simulink model "vf_controlled_3_phase_squirrel_cage"  (R2024a)
settings: Solver=VariableStepAuto  StartTime=0.0  StopTime=5  RelTol=1e-3
libraries: spsControlledVoltageSourceLib x3, simulink x2, spsAsynchronousMachineSIUnitsLib x1, spsGroundLib x1, sps_lib x1
settings Model: Creator=baileyraven  LastModifiedBy=baileyraven
settings SolverCC: ZeroCrossAlgorithm=Adaptive
settings OptimizationCC: ReuseModelBlockBuffer=off
settings DebuggingCC: IgnoredZcDiagnostic=none
settings RTWCC: GPUComputeCapability=3.5

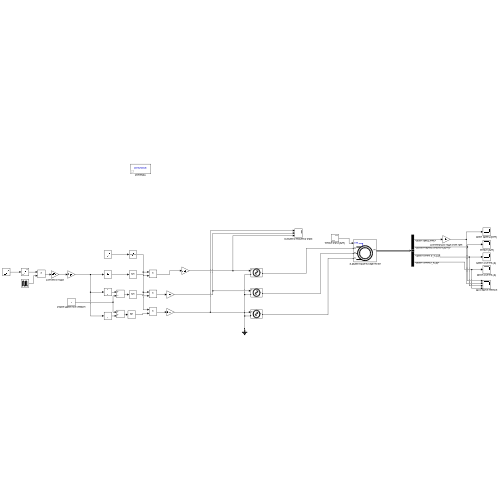
[thumbnail: Simulink's stored preview of the top-level diagram]
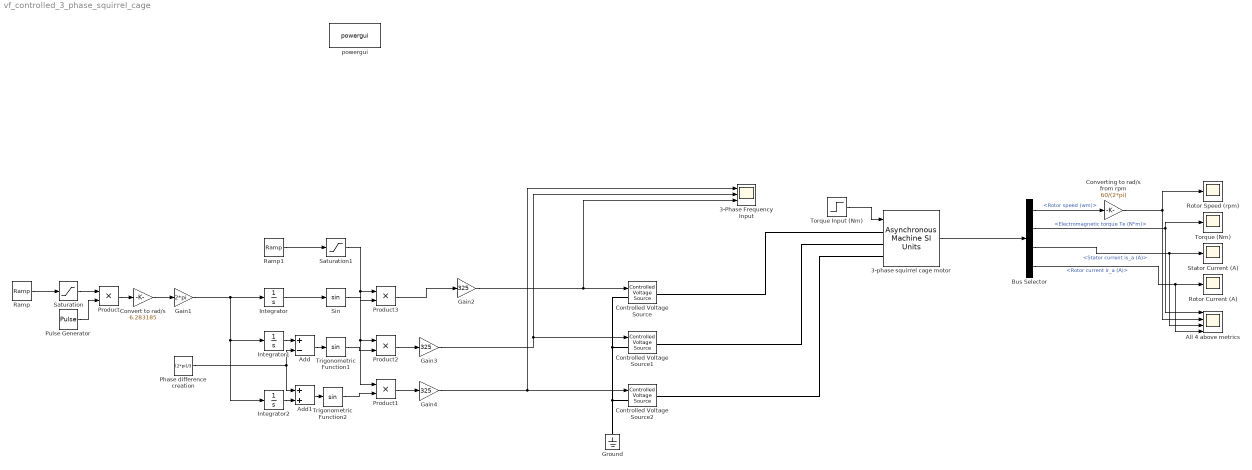
== system vf_controlled_3_phase_squirrel_cage ==
  " 3-phase squirrel cage motor" : spsAsynchronousMachineSIUnitsLib/Asynchronous Machine SI Units  RotorType=Squirrel-cage  PresetModel=No  MechanicalLoad=Torque Tm  ShowDetailedParameters=on  ReferenceFrame=Rotor  Units=SI  MeasurementBus=off  NominalParameters=[7460 281.69 50]  VoltageRatio=1  Stator=[0.8 0.009063]  Rotor=[0.8 0.009063]  Cage1=[0.4155 0.002066]  Cage2=[0.4168 0.0003495]  Lm=0.637  Mechanical=[0.1 0 2]  PolePairs=2  InitialConditions=[1 0 0 0 0 0 0 0]  SimulateSaturation=off  Saturation=[14.03593122, 27.81365428, 53.79336849, 72.68890987, 97.98006896, 148.6815601, 215.7428561, 302.9841135, 428.7778367 ; 230, 322, 414, 460, 506, 552, 598, 644, 690]  LoadFlowParameters=1492000  TsPowergui=0  TsBlock=-1  IterativeModel=Trapezoidal non iterative  IterativeDiscreteModel=Trapezoidal non iterative  Pmec=1.492e+006
  " Torque (Nm)" : Scope
  3-Phase Frequency Input : Scope  NumInputPorts=3
  Add : Sum  Inputs=+-
  Add1 : Sum
  All 4 above metrics : Scope  NumInputPorts=4
  Bus Selector : BusSelector  OutputSignals=Mechanical.Rotor speed (wm),Mechanical.Electromagnetic torque Te (N*m),Stator measurements.Stator current is_a (A),Rotor measurements.Rotor current ir_a (A)
  Controlled Voltage Source : spsControlledVoltageSourceLib/Controlled Voltage Source  Initialize=on  Source_Type=AC  Amplitude=0  Phase=0  Frequency=0  Measurements=None
  Controlled Voltage Source1 : spsControlledVoltageSourceLib/Controlled Voltage Source  Initialize=on  Source_Type=AC  Amplitude=0  Phase=0  Frequency=0  Measurements=None
  Controlled Voltage Source2 : spsControlledVoltageSourceLib/Controlled Voltage Source  Initialize=on  Source_Type=AC  Amplitude=0  Phase=0  Frequency=0  Measurements=None
  Convert to rad/s : Gain  Gain=6.283185
  Converting to rad/s from rpm : Gain  Gain=60/(2*pi)
  Gain1 : Gain  Gain=2*pi
  Gain2 : Gain  Gain=325
  Gain3 : Gain  Gain=325
  Gain4 : Gain  Gain=325
  Ground : spsGroundLib/Ground  LConnTagsString=a
  Integrator : Integrator
  Integrator1 : Integrator
  Integrator2 : Integrator
  Phase difference creation : Constant  Value=(2*pi)/3
  Product{,1..3} (4 alike) : Product
  Pulse Generator : DiscretePulseGenerator  PulseType=Time based  Period=0.0001  PulseWidth=5
  Ramp : simulink/Sources/Ramp  slope=90  start=0  InitialOutput=5
  Ramp1 : simulink/Sources/Ramp  slope=2  start=0  InitialOutput=0
  Rotor Current (A) : Scope
  Rotor Speed (rpm) : Scope
  Saturation : Saturate  UpperLimit=50  LowerLimit=5
  Saturation1 : Saturate  UpperLimit=1
  Sin : Trigonometry
  "Stator Current (A) " : Scope
  Torque Input (Nm) : Step  Time=1.5  After=49.89  SampleTime=0
  Trigonometric Function1 : Trigonometry
  Trigonometric Function2 : Trigonometry
  powergui : sps_lib/powergui  Priority=1  SimulationMode=Continuous  SampleTime=50e-6  frequency=60  Iterations=50  frequencyindice=0  Pbase=100e6  ErrMax=1e-4  UnitsV=kV  UnitsW=MW  buscounter=0  FunctionMessages=off  echomessages=off  EnableUseOfTLC=off  CurrentSourceSwitches=off  DisableSnubberDevices=off  DisableRonSwitches=off  DisableVfSwitches=off  DisplayEquations=off  AutomaticDiscreteSolvers=off  SolverType=Tustin/Backward Euler (TBE)  Interpol=off  ExternalGateDelay=off  methode=off  Ts=100  x0status=blocks  SPID=on  SwTol=0  HookPort=off  NonlinearTolerance=1e-4  nMaxIteration=100  ContinueOnMaxIteration=off  RestoreLinks=warning  ResistiveCurrentMeasurement=off  Frange=[0:2:500]  Ylog=off  Xlog=on  ShowGrid=off  save=off  variable=ZData  structure=0  ZoomFFT=off  StartTime=0.0  cycles=1  DisplayStyle=1  fundamental=60  FreqAxis=off  MaxFrequency=1000  frequencyindicesteady=1  RmsSteady=1  display=off
  wires:
  Ramp/1 -> Saturation/1
  Phase difference creation/1 -> Add/2, Add1/1
  Add/1 -> Trigonometric Function1/1
  Add1/1 -> Trigonometric Function2/1
  Integrator2/1 -> Add1/2
  Integrator1/1 -> Add/1
  Saturation/1 -> Product/1
  Sin/1 -> Product3/2
  Trigonometric Function1/1 -> Product2/2
  Integrator/1 -> Sin/1
  Trigonometric Function2/1 -> Product1/2
  Convert to rad/s/1 -> Gain1/1
  Gain1/1 -> Integrator/1, Integrator1/1, Integrator2/1
  Product/1 -> Convert to rad/s/1
  Pulse Generator/1 -> Product/2
  " 3-phase squirrel cage motor"/1 -> Bus Selector/1
  Converting to rad/s from rpm/1 -> All 4 above metrics/2, Rotor Speed (rpm)/1
  Torque Input (Nm)/1 -> " 3-phase squirrel cage motor"/1
  Product3/1 -> Gain2/1
  Product2/1 -> Gain3/1
  Product1/1 -> Gain4/1
  Ramp1/1 -> Saturation1/1
  Saturation1/1 -> Product3/1, Product2/1, Product1/1
  Bus Selector/1 -> Converting to rad/s from rpm/1  "<Rotor speed (wm)>"
  Bus Selector/2 -> " Torque (Nm)"/1, All 4 above metrics/1  "<Electromagnetic torque Te (N*m)>"
  Bus Selector/3 -> "Stator Current (A) "/1, All 4 above metrics/3  "<Stator current is_a (A)>"
  Bus Selector/4 -> Rotor Current (A)/1, All 4 above metrics/4  "<Rotor current ir_a (A)>"
  Gain4/1 -> 3-Phase Frequency Input/1, Controlled Voltage Source2/1
  Gain3/1 -> 3-Phase Frequency Input/2, Controlled Voltage Source1/1
  Gain2/1 -> 3-Phase Frequency Input/3, Controlled Voltage Source/1
  connections:
  Controlled Voltage Source/RConn1 -- " 3-phase squirrel cage motor"/LConn1
  Controlled Voltage Source2/RConn1 -- " 3-phase squirrel cage motor"/LConn3
  Controlled Voltage Source1/RConn1 -- " 3-phase squirrel cage motor"/LConn2
  Controlled Voltage Source/LConn1 -- Controlled Voltage Source1/LConn1 -- Controlled Voltage Source2/LConn1 -- Ground/LConn1
